simulink model "test_generator"  (R2021b)
settings: Solver=VariableStepAuto  StartTime=0.0  StopTime=inf  FixedStep=.01  RelTol=1e-3
values from neighbouring files (symbols this model uses):
  c = param(21)    [get_full_state.m]
  k_line = param(19)    [get_full_state.m]
  r = state(12)    [get_ac_forces_moments.m]    (also in get_full_state.m = param(17))
undefined symbols (not defined in the file or in its folder): InitTheta, InitThetaDot, moi, theta_0
settings Model: PacingRate=16  Creator=austm  LastModifiedBy=austm
settings SFSimCC: SimTargetLang=C++

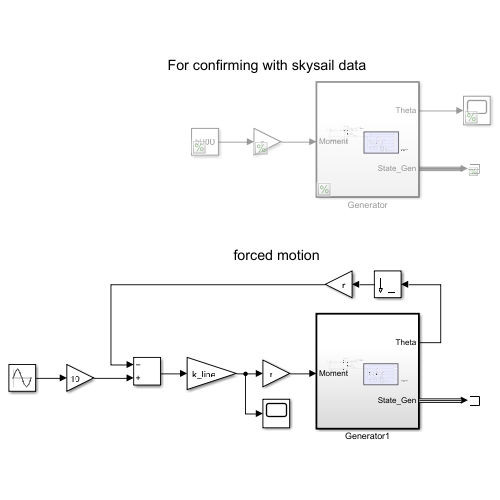
[thumbnail: Simulink's stored preview of the top-level diagram]
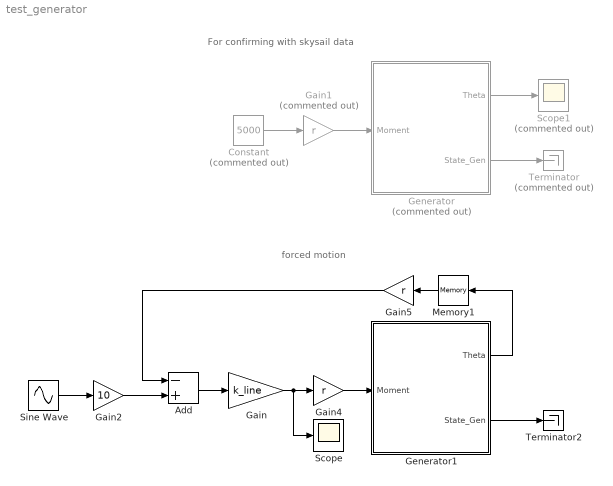
== system test_generator ==
  note: For confirming with skysail data
  note: forced motion
  Add : Sum  Inputs=-+
  Constant : Constant  Commented=on  Value=5000
  Gain : Gain  Gain=k_line
  Gain1 : Gain  Commented=on  Gain=r
  Gain2 : Gain  Gain=10
  Gain4 : Gain  Gain=r
  Gain5 : Gain  Gain=r
  Generator : Subsystem  Commented=on  TreatAsAtomicUnit=on
  Generator1 : Subsystem  TreatAsAtomicUnit=on
  Memory1 : Memory
  Scope : Scope
  Scope1 : Scope  Commented=on
  Sine Wave : Sin  Bias=-1  Frequency=2*pi*.04  Phase=90*pi/180  SampleTime=0
  Terminator : Terminator  Commented=on
  Terminator2 : Terminator
  wires:
  Sine Wave/1 -> Gain2/1
  Gain1/1 -> Generator/1(Moment)
  Generator/2(State_Gen) -> Terminator/1
  Generator/1(Theta) -> Scope1/1
  Gain2/1 -> Add/2
  Add/1 -> Gain/1
  Constant/1 -> Gain1/1
  Gain/1 -> Scope/1, Gain4/1
  Gain5/1 -> Add/1
  Generator1/1(Theta) -> Memory1/1
  Gain4/1 -> Generator1/1(Moment)
  Memory1/1 -> Gain5/1
  Generator1/2(State_Gen) -> Terminator2/1

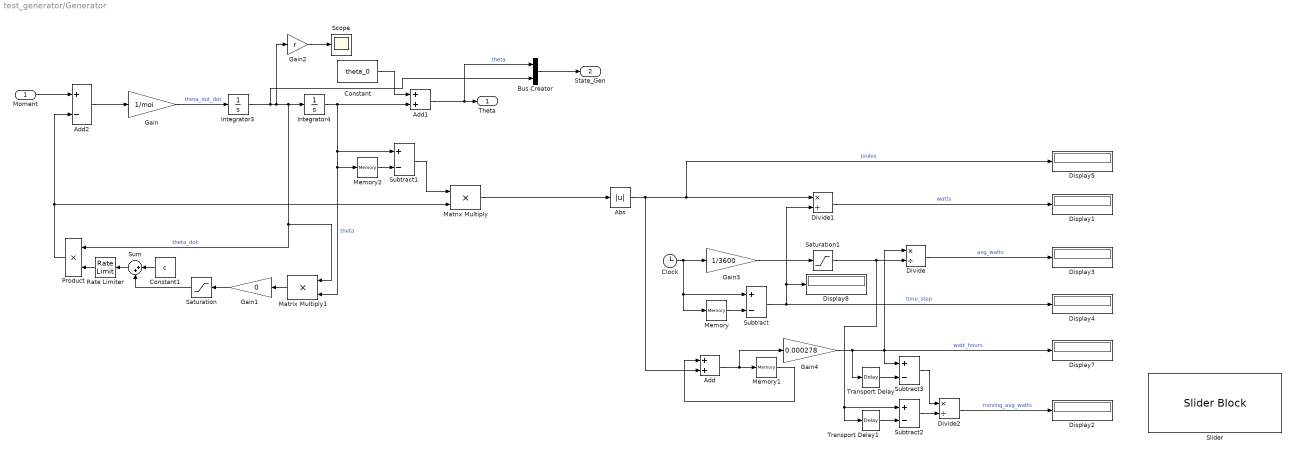
== system test_generator/Generator ==
  Moment : Inport
  Abs : Abs
  Add : Sum
  Add1 : Sum
  Add2 : Sum  Inputs=+-
  Bus Creator : BusCreator  Inputs=2
  Clock : Clock
  Constant : Constant  Value=theta_0
  Constant1 : Constant  Value=c
  Display{1..5,7..8} (7 alike) : Display
  Divide : Product  Inputs=*/
  Divide1 : Product  Inputs=*/
  Divide2 : Product  Inputs=*/
  Gain : Gain  Gain=1/moi
  Gain1 : Gain  Gain=0
  Gain2 : Gain  Gain=r
  Gain3 : Gain  Gain=1/3600
  Gain4 : Gain  Gain=0.000278
  Integrator3 : Integrator  InitialCondition=InitThetaDot
  Integrator4 : Integrator  InitialCondition=InitTheta
  Matrix Multiply : Product
  Matrix Multiply1 : Product
  Memory : Memory  InitialCondition=-.001
  Memory1 : Memory
  Memory2 : Memory
  Product : Product
  Rate Limiter : RateLimiter  RisingSlewLimit=10  FallingSlewLimit=-10  SampleTimeMode=inherited
  Saturation : Saturate  UpperLimit=c  LowerLimit=-c
  Saturation1 : Saturate  UpperLimit=inf  LowerLimit=0.00001
  Scope : Scope
  Slider : SliderBlock  ScaleMax=50
  Subtract{,1..3} (4 alike) : Sum  Inputs=+-
  Sum : Sum  Inputs=|++
  Transport Delay : TransportDelay  DelayTime=30  BufferSize=5120
  Transport Delay1 : TransportDelay  DelayTime=30  BufferSize=5120
  Theta : Outport
  State_Gen : Outport  Port=2
  wires:
  Moment/1 -> Add2/1
  Constant/1 -> Add1/1
  Add2/1 -> Gain/1
  Gain/1 -> Integrator3/1  "theta_dot_dot"
  Integrator3/1 -> Bus Creator/2, Gain2/1, Product/1, Matrix Multiply1/1, Integrator4/1  "theta_dot"
  Integrator4/1 -> Add1/2, Matrix Multiply1/2, Memory2/1, Subtract1/1  "theta"
  Add1/1 -> Bus Creator/1, Theta/1  "theta"
  Subtract1/1 -> Matrix Multiply/1
  Abs/1 -> Display5/1, Divide1/1, Add/2  "joules"
  Matrix Multiply1/1 -> Gain1/1
  Product/1 -> Matrix Multiply/2, Add2/2
  Clock/1 -> Memory/1, Subtract/1, Gain3/1
  Gain3/1 -> Saturation1/1
  Divide/1 -> Display3/1  "avg_watts"
  Memory/1 -> Subtract/2
  Subtract/1 -> Divide1/2, Display8/1, Display4/1  "time_step"
  Divide1/1 -> Display1/1  "watts"
  Matrix Multiply/1 -> Abs/1
  Add/1 -> Memory1/1, Gain4/1
  Memory1/1 -> Add/1
  Gain4/1 -> Display7/1, Subtract3/1, Divide/1, Transport Delay/1  "watt_hours"
  Memory2/1 -> Subtract1/2
  Sum/1 -> Rate Limiter/1
  Constant1/1 -> Sum/1
  Gain1/1 -> Saturation/1
  Rate Limiter/1 -> Product/2
  Saturation/1 -> Sum/2
  Transport Delay1/1 -> Subtract2/2
  Subtract2/1 -> Divide2/2
  Transport Delay/1 -> Subtract3/2
  Subtract3/1 -> Divide2/1
  Divide2/1 -> Display2/1  "moving_avg_watts"
  Saturation1/1 -> Divide/2, Subtract2/1, Transport Delay1/1
  Bus Creator/1 -> State_Gen/1
  Gain2/1 -> Scope/1

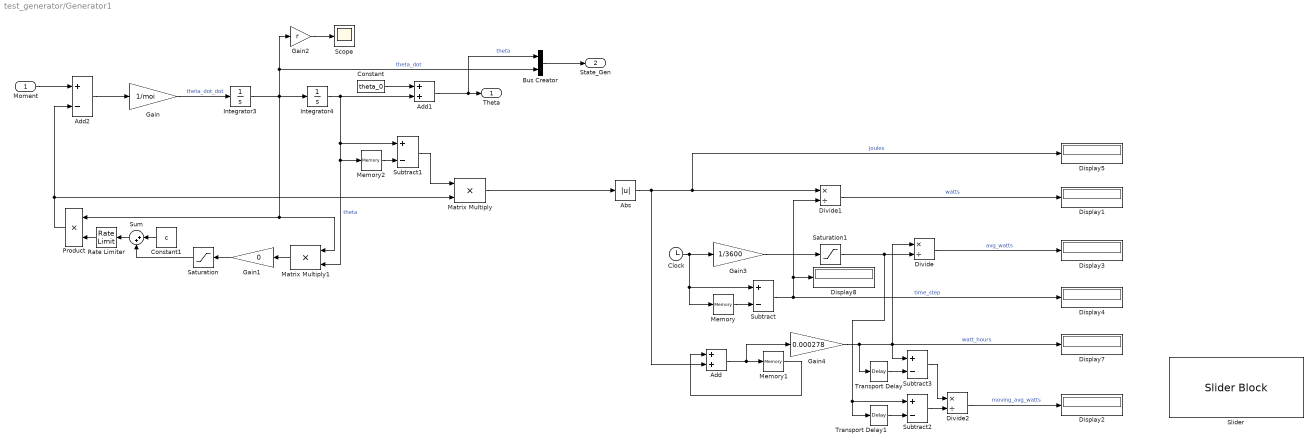
== system test_generator/Generator1 ==
  Moment : Inport
  Abs : Abs
  Add : Sum
  Add1 : Sum
  Add2 : Sum  Inputs=+-
  Bus Creator : BusCreator  Inputs=2
  Clock : Clock
  Constant : Constant  Value=theta_0
  Constant1 : Constant  Value=c
  Display{1..5,7..8} (7 alike) : Display
  Divide : Product  Inputs=*/
  Divide1 : Product  Inputs=*/
  Divide2 : Product  Inputs=*/
  Gain : Gain  Gain=1/moi
  Gain1 : Gain  Gain=0
  Gain2 : Gain  Gain=r
  Gain3 : Gain  Gain=1/3600
  Gain4 : Gain  Gain=0.000278
  Integrator3 : Integrator
  Integrator4 : Integrator
  Matrix Multiply : Product
  Matrix Multiply1 : Product
  Memory : Memory  InitialCondition=-.001
  Memory1 : Memory
  Memory2 : Memory
  Product : Product
  Rate Limiter : RateLimiter  RisingSlewLimit=10  FallingSlewLimit=-10  SampleTimeMode=inherited
  Saturation : Saturate  UpperLimit=c  LowerLimit=-c
  Saturation1 : Saturate  UpperLimit=inf  LowerLimit=0.00001
  Scope : Scope
  Slider : SliderBlock  ScaleMax=400
  Subtract{,1..3} (4 alike) : Sum  Inputs=+-
  Sum : Sum  Inputs=|++
  Transport Delay : TransportDelay  DelayTime=60  BufferSize=5120
  Transport Delay1 : TransportDelay  DelayTime=60  BufferSize=5120
  Theta : Outport
  State_Gen : Outport  Port=2
  wires:
  Moment/1 -> Add2/1
  Constant/1 -> Add1/1
  Add2/1 -> Gain/1
  Gain/1 -> Integrator3/1  "theta_dot_dot"
  Integrator3/1 -> Integrator4/1, Matrix Multiply1/1, Product/1, Bus Creator/2, Gain2/1  "theta_dot"
  Integrator4/1 -> Add1/2, Matrix Multiply1/2, Memory2/1, Subtract1/1  "theta"
  Add1/1 -> Bus Creator/1, Theta/1  "theta"
  Subtract1/1 -> Matrix Multiply/1
  Abs/1 -> Display5/1, Divide1/1, Add/2  "joules"
  Matrix Multiply1/1 -> Gain1/1
  Product/1 -> Matrix Multiply/2, Add2/2
  Clock/1 -> Memory/1, Subtract/1, Gain3/1
  Gain3/1 -> Saturation1/1
  Divide/1 -> Display3/1  "avg_watts"
  Memory/1 -> Subtract/2
  Subtract/1 -> Divide1/2, Display8/1, Display4/1  "time_step"
  Divide1/1 -> Display1/1  "watts"
  Matrix Multiply/1 -> Abs/1
  Add/1 -> Memory1/1, Gain4/1
  Memory1/1 -> Add/1
  Gain4/1 -> Display7/1, Subtract3/1, Divide/1, Transport Delay/1  "watt_hours"
  Memory2/1 -> Subtract1/2
  Sum/1 -> Rate Limiter/1
  Constant1/1 -> Sum/1
  Gain1/1 -> Saturation/1
  Rate Limiter/1 -> Product/2
  Saturation/1 -> Sum/2
  Transport Delay1/1 -> Subtract2/2
  Subtract2/1 -> Divide2/2
  Transport Delay/1 -> Subtract3/2
  Subtract3/1 -> Divide2/1
  Divide2/1 -> Display2/1  "moving_avg_watts"
  Saturation1/1 -> Divide/2, Subtract2/1, Transport Delay1/1
  Bus Creator/1 -> State_Gen/1
  Gain2/1 -> Scope/1
